simulink model "modele_helice"  (R2025b)
settings: Solver=VariableStepAuto  StartTime=0.0  StopTime=50  RelTol=1e-3
values from neighbouring files (symbols this model uses):
  Axy = 0.0    (= 0)    [PropKtKq.m]
  Cxy = 0.0    (= 0)    [PropKtKq.m]
  D = 0.0    (= 0)    [PropKtKq.m]
  th = 0.0    (= 0)    [Hulldyn.m]    (also in PropKtKq.m; variables_procom.m = 0.214)
  wh = 0.0    (= 0)    [Hulldyn.m]    (also in PropKtKq.m)
  x = 0.0    (= 0)    [PropKtKq.m]
  y = 0.0    (= 0)    [PropKtKq.m]
settings Model: Creator=leagr  LastModifiedBy=f23berge

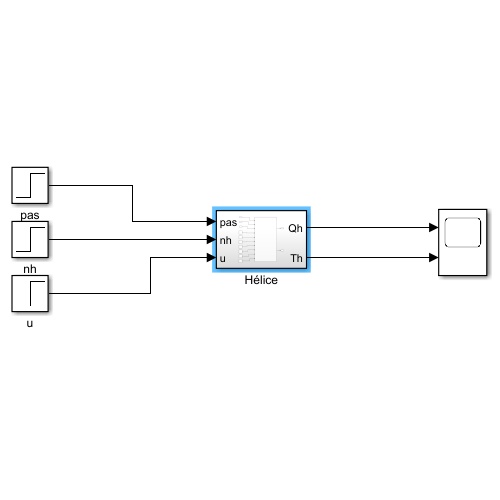
[thumbnail: Simulink's stored preview of the top-level diagram]
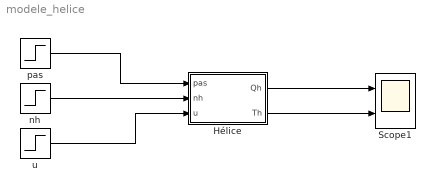
== system modele_helice ==
  Hélice : Subsystem
  Scope1 : Scope  NumInputPorts=2
      settings: ActiveDisplayYMinimum=-290396.18557121255  ActiveDisplayYMaximum=2.6135656701409137E+6
  nh : Step  After=80  SampleTime=0
  pas : Step  After=0  SampleTime=0
  u : Step  After=5  SampleTime=0
  wires:
  Hélice/1(Qh) -> Scope1/1
  Hélice/2(Th) -> Scope1/2
  u/1 -> Hélice/3(u)
  nh/1 -> Hélice/2(nh)
  pas/1 -> Hélice/1(pas)

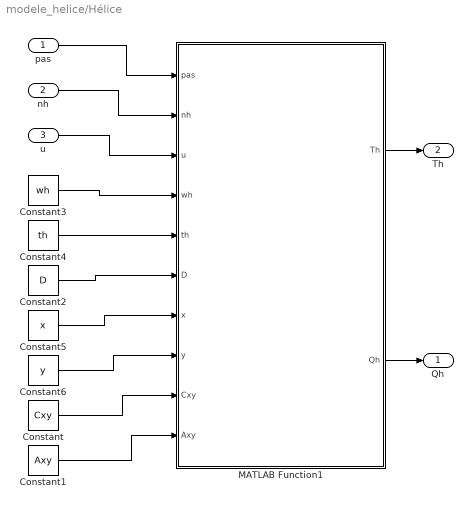
== system modele_helice/Hélice ==
  pas : Inport
  nh : Inport  Port=2
  u : Inport  Port=3
  Constant : Constant  Value=Cxy
  Constant1 : Constant  Value=Axy
  Constant2 : Constant  Value=D
  Constant3 : Constant  Value=wh
  Constant4 : Constant  Value=th
  Constant5 : Constant  Value=x
  Constant6 : Constant  Value=y
  MATLAB Function1 : MATLAB Function  TreatAsAtomicUnit=on
  Qh : Outport
  Th : Outport  Port=2
  wires:
  pas/1 -> MATLAB Function1/1(pas)
  nh/1 -> MATLAB Function1/2(nh)
  Constant/1 -> MATLAB Function1/9(Cxy)
  u/1 -> MATLAB Function1/3(u)
  Constant3/1 -> MATLAB Function1/4(wh)
  Constant4/1 -> MATLAB Function1/5(th)
  Constant1/1 -> MATLAB Function1/10(Axy)
  Constant2/1 -> MATLAB Function1/6(D)
  Constant5/1 -> MATLAB Function1/7(x)
  Constant6/1 -> MATLAB Function1/8(y)
  MATLAB Function1/2(Qh) -> Qh/1
  MATLAB Function1/1(Th) -> Th/1

== matlab function modele_helice/Hélice/MATLAB Function1 ==
  data: pas input; nh input; u input; Th output; Qh output; wh input; th input; D input; x input; y input; Cxy input; Axy input
function [Th,Qh]= fcn(pas, nh, u, wh, th ,D, x, y, Cxy, Axy)
    
    % /!\ nh en rad/s

    rho = 1025; % Masse volumique de l'eau

    % Coefficient d'avance et rapport P/D
    J = u*(1-wh)/(D*nh);
    P_D = pas/D;
        
    % Calcul des coefficients Kt et Kq pour ce point de fonctionnement
    if nh < 1e-6
        Kt = 0;
        Kq = 0;
    else
        Kt = dot(Axy, P_D.^x .* J.^y);
        Kq = dot(Cxy, P_D.^x .* J.^y);
    end
    
    % Calcul de la poussée
    Th = (1-th)*Kt*rho*D^4*nh^2;
    Qh = Kq*rho*D^5*nh^2;

end
